simulink model "controller"  (R2017b)
settings: Solver=VariableStepAuto  StartTime=0.0  StopTime=10.0  RelTol=1e-3
undefined symbols (not defined in the file): Kd, Ki, Kp
settings Model: Creator=stankasa  LastModifiedBy=stankasa

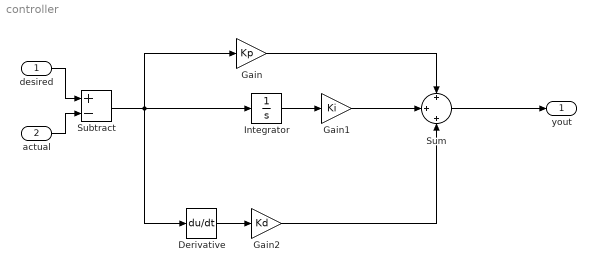
== system controller ==
  desired : Inport
  actual : Inport  Port=2
  Derivative : Derivative  CoefficientInTFapproximation=0
  Gain : Gain  Gain=Kp
  Gain1 : Gain  Gain=Ki
  Gain2 : Gain  Gain=Kd
  Integrator : Integrator
  Subtract : Sum  Inputs=+-
  Sum : Sum  Inputs=+|+|+
  yout : Outport
  wires:
  desired/1 -> Subtract/1
  actual/1 -> Subtract/2
  Subtract/1 -> Gain/1, Integrator/1, Derivative/1
  Derivative/1 -> Gain2/1
  Integrator/1 -> Gain1/1
  Gain/1 -> Sum/1
  Gain1/1 -> Sum/2
  Gain2/1 -> Sum/3
  Sum/1 -> yout/1
